simulink model "ASMC_sim_CSEI_FTESO"  (R2022a)
settings: Solver=ode4  StartTime=0.0  StopTime=T_final  FixedStep=Ts  RelTol=1e-3
values from neighbouring files (symbols this model uses):
  ASMC_enabled = 1    [ASMC_ESO_sim_CSEI_Scripts.m]    (also in ASMC_FTESO_sim_CSEI_Scripts.m)
  BL = [20 10 10]    [ASMC_ESO_sim_CSEI_Scripts.m]    (also in ASMC_FTESO_sim_CSEI_Scripts.m; SMC_ESO_sim_CSEI_Scripts.m; SMC_sim_CSEI_Scripts.m)
  Control_allocation = 1    [ASMC_ESO_sim_CSEI_Scripts.m]    (also in ASMC_FTESO_sim_CSEI_Scripts.m; SMC_ESO_sim_CSEI_Scripts.m; SMC_sim_CSEI_Scripts.m)
  current = [0;0]    [ASMC_ESO_sim_CSEI_Scripts.m]    (also in ASMC_FTESO_sim_CSEI_Scripts.m; Berthing_Control_PID_CSEI_Scripts.m; Position_Control_PID_CSEI_Scripts.m; Position_Control_PID_CSEI_Scripts_released.m)
  Disturbance_enabled = 1    [ASMC_ESO_sim_CSEI_Scripts.m]    (also in ASMC_FTESO_sim_CSEI_Scripts.m; SMC_ESO_sim_CSEI_Scripts.m)
  disturbance_type = 0    [ASMC_ESO_sim_CSEI_Scripts.m]    (also in ASMC_FTESO_sim_CSEI_Scripts.m = 2)
  ESO_enabled = 1    [ASMC_ESO_sim_CSEI_Scripts.m]    (also in ASMC_FTESO_sim_CSEI_Scripts.m; SMC_ESO_sim_CSEI_Scripts.m = 0)
  ESO_type = 2    [ASMC_FTESO_sim_CSEI_Scripts.m]
  ESO_type_enabled = 1    [ASMC_FTESO_sim_CSEI_Scripts.m]
  k1_init = 0.1*[5;5;10]    [ASMC_ESO_sim_CSEI_Scripts.m]    (also in ASMC_FTESO_sim_CSEI_Scripts.m)
  k2 = [5;5;5]    [ASMC_ESO_sim_CSEI_Scripts.m]    (also in ASMC_FTESO_sim_CSEI_Scripts.m)
  k3 = 0.05*[10; 20; 50]    [ASMC_ESO_sim_CSEI_Scripts.m]    (also in ASMC_FTESO_sim_CSEI_Scripts.m)
  k_min = 1    [ASMC_ESO_sim_CSEI_Scripts.m]    (also in ASMC_FTESO_sim_CSEI_Scripts.m)
  K_SMC = [20 20 50]    [ASMC_ESO_sim_CSEI_Scripts.m]    (also in ASMC_FTESO_sim_CSEI_Scripts.m; SMC_ESO_sim_CSEI_Scripts.m; SMC_sim_CSEI_Scripts.m)
  lamda = [5.0 5.0 10]    [ASMC_ESO_sim_CSEI_Scripts.m]    (also in ASMC_FTESO_sim_CSEI_Scripts.m; SMC_ESO_sim_CSEI_Scripts.m; SMC_sim_CSEI_Scripts.m)
  mu = [0.005; 0.005; 0.005]    [ASMC_ESO_sim_CSEI_Scripts.m]    (also in ASMC_FTESO_sim_CSEI_Scripts.m)
  option = 0    [ASMC_ESO_sim_CSEI_Scripts.m]    (also in ASMC_FTESO_sim_CSEI_Scripts.m; SMC_ESO_sim_CSEI_Scripts.m = 1; SMC_sim_CSEI_Scripts.m = 1)
  psi_ref = 40    [ASMC_ESO_sim_CSEI_Scripts.m]    (also in ASMC_FTESO_sim_CSEI_Scripts.m; SMC_ESO_sim_CSEI_Scripts.m; SMC_sim_CSEI_Scripts.m)
  tau_max = 20*[3; 3; 3]    [ASMC_ESO_sim_CSEI_Scripts.m]    (also in ASMC_FTESO_sim_CSEI_Scripts.m; SMC_ESO_sim_CSEI_Scripts.m; SMC_sim_CSEI_Scripts.m)
  v_max = 10    [ASMC_ESO_sim_CSEI_Scripts.m]    (also in ASMC_FTESO_sim_CSEI_Scripts.m; Position_Control_PID_CSEI_Scripts.m = 2; Position_Control_PID_CSEI_Scripts_released.m = 2; SMC_ESO_sim_CSEI_Scripts.m)
  w0 = 60    [ASMC_ESO_sim_CSEI_Scripts.m]    (also in ASMC_FTESO_sim_CSEI_Scripts.m; SMC_ESO_sim_CSEI_Scripts.m)
  w0_FTESO = 10    [ASMC_FTESO_sim_CSEI_Scripts.m]
  w_d = 0.5    [ASMC_ESO_sim_CSEI_Scripts.m]    (also in ASMC_FTESO_sim_CSEI_Scripts.m; SMC_ESO_sim_CSEI_Scripts.m; SMC_sim_CSEI_Scripts.m)
  x0 = zeros(6,1)    [Berthing_Control_PID_CSEI_Scripts.m]    (also in Position_Control_PID_CSEI_Scripts.m; Position_Control_PID_CSEI_Scripts_released.m; Waypoint_Control_PID_CSEI_Scripts.m; Waypoint_Control_PID_CSEI_Scripts_LLA.m)
  x_ref = 7    [ASMC_ESO_sim_CSEI_Scripts.m]    (also in ASMC_FTESO_sim_CSEI_Scripts.m; SMC_ESO_sim_CSEI_Scripts.m; SMC_sim_CSEI_Scripts.m)
  y_ref = 7    [ASMC_ESO_sim_CSEI_Scripts.m]    (also in ASMC_FTESO_sim_CSEI_Scripts.m; SMC_ESO_sim_CSEI_Scripts.m; SMC_sim_CSEI_Scripts.m)
  zeta_d = 1    [ASMC_ESO_sim_CSEI_Scripts.m]    (also in ASMC_FTESO_sim_CSEI_Scripts.m; SMC_ESO_sim_CSEI_Scripts.m; SMC_sim_CSEI_Scripts.m)
undefined symbols (not defined in the file or in its folder): sigbuilder_block
libraries: simulink_extras x5
(part 1 of 2)
settings Model: Creator=ADMIN  LastModifiedBy=ADMIN

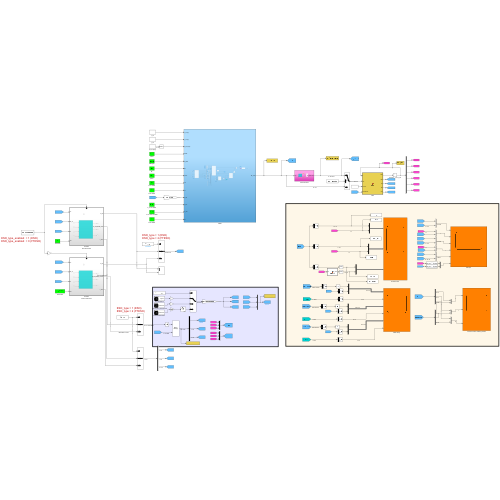
[thumbnail: Simulink's stored preview of the top-level diagram]
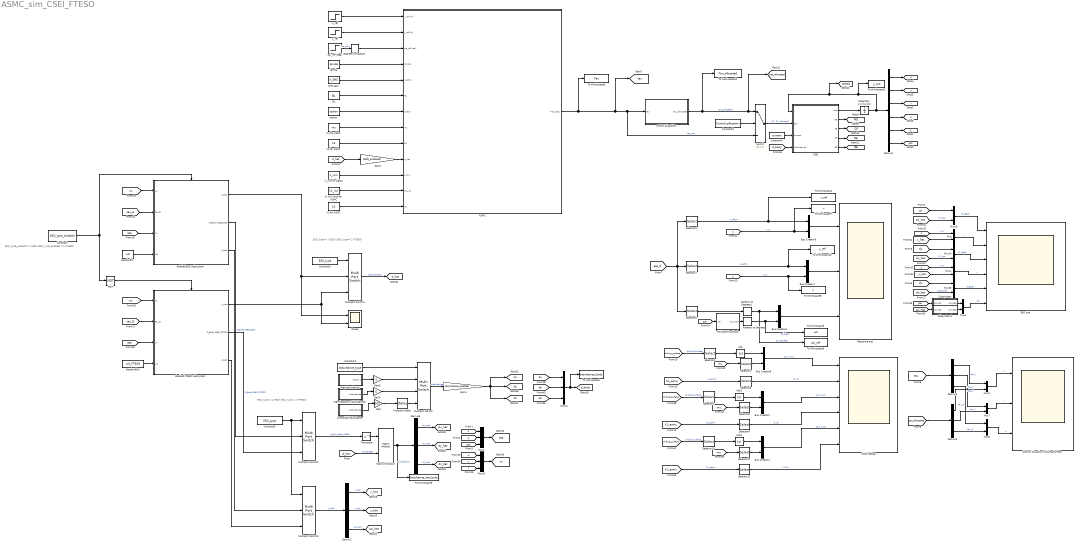
== system ASMC_sim_CSEI_FTESO ==
  note: ESO_type = 1 (ESO)
      | ESO_type = 2 (FTESO)
  note: ESO_type = 1 (ESO)
      | ESO_type = 2 (FTESO)
  note: ESO_type_enabled = 1 (ESO)
      | ESO_type_enabled = 0 (FTESO)
  ASMC : Subsystem
  ASMC debug : Scope  NumInputPorts=6
  Abs : Abs  SaturateOnIntegerOverflow=off
  Abs1 : Abs  SaturateOnIntegerOverflow=off
  Abs2 : Abs  SaturateOnIntegerOverflow=off
  BL : Constant  Value=BL
  Bandwidth : Constant  Value=w0
  Bandwidth2 : Constant  Value=w0_FTESO
  Bus Creator{1..6} (6 alike) : BusCreator  Inputs=2
  CSEI : MATLAB Function  TreatAsAtomicUnit=on
  Constant : Constant  Value=ESO_type_enabled
  Constant1 : Constant  Value=disturbance_type
  Constant2 : Constant  Value=ESO_type
  Constant3 : Constant  Value=Control_allocation
  Constant4 : Constant  Value=current
  Constant5 : Constant  Value=ESO_type
  Control Alocation & Sliding Surface : Scope  NumInputPorts=3
  Degrees to Radians : simulink_extras/Transformations/Degrees to Radians
  Demux1 : Demux  Outputs=6
  Demux{2..3,5,8} (4 alike) : Demux  Outputs=3
  ESO plot : Scope  NumInputPorts=6
  Enabled ESO Subsystem : Subsystem  TreatAsAtomicUnit=on
  Enabled FTESO Subsystem : Subsystem  TreatAsAtomicUnit=on
  Gain : Gain  Gain=100
  Gain1 : Gain  Gain=Disturbance_enabled
  Gain2 : Gain  Gain=ESO_enabled
  Gain3 : Gain  Gain=6
  Gain5 : Gain  Gain=5
  "Integrator : u;v;r;x;y;psi" : Integrator  InitialCondition=x0
  MATLAB Function3 : MATLAB Function  TreatAsAtomicUnit=on
  Matrix Multiply3 : Product  Multiplication=Matrix(*)
  Multiport Switch : MultiPortSwitch  SaturateOnIntegerOverflow=off  InputSameDT=off
  Multiport Switch1 : MultiPortSwitch  Inputs=2  SaturateOnIntegerOverflow=off  InputSameDT=off
  Multiport Switch2 : MultiPortSwitch  Inputs=2  SaturateOnIntegerOverflow=off  InputSameDT=off
  Multiport Switch3 : MultiPortSwitch  Inputs=2  SaturateOnIntegerOverflow=off  InputSameDT=off
  Mux{,1,3..4,7..8,14..16} (9 alike) : Mux  Inputs=2
  Mux10 : Mux  Inputs=3
  Mux11 : Mux  Inputs=3
  Mux2 : Mux  Inputs=3
  NOT : Logic  Operator=NOT  IconShape=distinctive  AllPortsSameDT=off  OutDataTypeStr=boolean
  Radians to Degrees : simulink_extras/Transformations/Radians to Degrees
  Radians to Degrees1 : simulink_extras/Transformations/Radians to Degrees
  Response plot : Scope  NumInputPorts=3
  SMC gain : Constant  Value=K_SMC
  Scope : Scope  NumInputPorts=2
  Selector1 : Selector  InputPortWidth=3  IndexOptions=Index vector (dialog)  Indices=1  OutputSizes=1
  Selector10 : Selector  InputPortWidth=3  IndexOptions=Index vector (dialog)  Indices=3  OutputSizes=1
  Selector11 : Selector  InputPortWidth=3  IndexOptions=Index vector (dialog)  Indices=3  OutputSizes=1
  Selector12 : Selector  InputPortWidth=3  IndexOptions=Index vector (dialog)  Indices=3  OutputSizes=1
  Selector2 : Selector  InputPortWidth=3  IndexOptions=Index vector (dialog)  Indices=1  OutputSizes=1
  Selector3 : Selector  InputPortWidth=3  IndexOptions=Index vector (dialog)  Indices=1  OutputSizes=1
  Selector4 : Selector  InputPortWidth=3  IndexOptions=Index vector (dialog)  Indices=2  OutputSizes=1
  Selector5 : Selector  InputPortWidth=3  IndexOptions=Index vector (dialog)  Indices=[3]  OutputSizes=1
  Selector6 : Selector  InputPortWidth=3  IndexOptions=Index vector (dialog)  Indices=[1]  OutputSizes=1
  Selector7 : Selector  InputPortWidth=3  IndexOptions=Index vector (dialog)  Indices=[2]  OutputSizes=1
  Selector8 : Selector  InputPortWidth=3  IndexOptions=Index vector (dialog)  Indices=2  OutputSizes=1
  Selector9 : Selector  InputPortWidth=3  IndexOptions=Index vector (dialog)  Indices=2  OutputSizes=1
  Subsystem : Subsystem
  Subsystem1 : Subsystem
  Switch : Switch  Criteria=u2 > Threshold  SaturateOnIntegerOverflow=off  InputSameDT=off
  To Workspace1 : ToWorkspace  VariableName=disturbance_body  SampleTime=-1
  To Workspace10 : ToWorkspace  VariableName=y_ref  SampleTime=-1
  To Workspace12 : ToWorkspace  VariableName=Tau_allocated  SampleTime=-1
  To Workspace2 : ToWorkspace  VariableName=y_out  SampleTime=-1
  To Workspace3 : ToWorkspace  VariableName=psi  SampleTime=-1
      settings: Save2DSignal=2-D array (concatenate along first dimension)
  To Workspace4 : ToWorkspace  VariableName=x_ref  SampleTime=-1
  To Workspace5 : ToWorkspace  VariableName=psi_ref  SampleTime=-1
  To Workspace6 : ToWorkspace  VariableName=Tau  SampleTime=-1
  To Workspace7 : ToWorkspace  VariableName=x  SampleTime=-1
      settings: Save2DSignal=2-D array (concatenate along first dimension)
  To Workspace8 : ToWorkspace  VariableName=y  SampleTime=-1
  To Workspace9 : ToWorkspace  VariableName=disturbance_hat_body  SampleTime=-1
  Transport Delay : TransportDelay  DelayTime=20
  Transpose : Math  Operator=transpose
  control allocation : Subsystem
  high-frequency disturbances : Subsystem  Tag=STV Subsys  LoadFcn=sigbuilder_block('load');  StartFcn=sigbuilder_block('start');  StopFcn=sigbuilder_block('stop');  ClipboardFcn=sigbuilder_block('clipboard');  mask(Sigbuilder block){tuvar=[0:10]}
      mask help: Simulink:masks:SigbuilderBlock_MD
      mask init:
      | if ~strcmp(get_param(bdroot(gcbh),'SimulationStatus'),'stopped') tuvar = sigbuilder_block('maskInit'); end
      settings: CopyFcn=sigbuilder_block('copy');  DeleteFcn=sigbuilder_block('delete');  ModelCloseFcn=sigbuilder_block('modelClose');  PreSaveFcn=sigbuilder_block('preSave');  PauseFcn=sigbuilder_block('pause');  ContinueFcn=sigbuilder_block('continue');  NameChangeFcn=sigbuilder_block('namechange');  OpenFcn=sigbuilder_block('open',[437.6 199.2 550.4 400 ]);  CloseFcn=sigbuilder_block('close');
      mask Display: plot(0, 0, 100, 100,[2, 2, 32, 32, 2], [68, 8, 8, 68, 68],[32, 2], [38, 38], [32, 19, 2],[53, 60, 44], [32, 17, 17, 2],[16, 16, 31, 31]);txt = getActiveGroup(gcbh);text(2, 100, txt,'verticalAlignment', 'top');
  k1 init value for ASMC : Constant  Value=k1_init
  k2 for ASMC : Constant  Value=k2
  k3 for ASMC : Constant  Value=k3
  k_min for ASMC : Constant  Value=k_min
  lamda : Constant  Value=lamda
  mu for ASMC : Constant  Value=mu
  option : Constant  Value=option
  psi_ref (deg) : Step  Time=10  After=psi_ref  SampleTime=0
  sinosoidal disturbance : Subsystem  Tag=STV Subsys  LoadFcn=sigbuilder_block('load');  StartFcn=sigbuilder_block('start');  StopFcn=sigbuilder_block('stop');  ClipboardFcn=sigbuilder_block('clipboard');  mask(Sigbuilder block){tuvar=[0:10]}
      mask help: Simulink:masks:SigbuilderBlock_MD
      mask init:
      | if ~strcmp(get_param(bdroot(gcbh),'SimulationStatus'),'stopped') tuvar = sigbuilder_block('maskInit'); end
      settings: CopyFcn=sigbuilder_block('copy');  DeleteFcn=sigbuilder_block('delete');  ModelCloseFcn=sigbuilder_block('modelClose');  PreSaveFcn=sigbuilder_block('preSave');  PauseFcn=sigbuilder_block('pause');  ContinueFcn=sigbuilder_block('continue');  NameChangeFcn=sigbuilder_block('namechange');  OpenFcn=sigbuilder_block('open',[437.6 199.2 550.4 400 ]);  CloseFcn=sigbuilder_block('close');
      mask Display: plot(0, 0, 100, 100,[2, 2, 32, 32, 2], [68, 8, 8, 68, 68],[32, 2], [38, 38], [32, 19, 2],[53, 60, 44], [32, 17, 17, 2],[16, 16, 31, 31]);txt = getActiveGroup(gcbh);text(2, 100, txt,'verticalAlignment', 'top');
  step disturbance : Subsystem  Tag=STV Subsys  LoadFcn=sigbuilder_block('load');  StartFcn=sigbuilder_block('start');  StopFcn=sigbuilder_block('stop');  ClipboardFcn=sigbuilder_block('clipboard');  mask(Sigbuilder block){tuvar=[0:10]}
      mask help: Simulink:masks:SigbuilderBlock_MD
      mask init:
      | if ~strcmp(get_param(bdroot(gcbh),'SimulationStatus'),'stopped') tuvar = sigbuilder_block('maskInit'); end
      settings: CopyFcn=sigbuilder_block('copy');  DeleteFcn=sigbuilder_block('delete');  ModelCloseFcn=sigbuilder_block('modelClose');  PreSaveFcn=sigbuilder_block('preSave');  PauseFcn=sigbuilder_block('pause');  ContinueFcn=sigbuilder_block('continue');  NameChangeFcn=sigbuilder_block('namechange');  OpenFcn=sigbuilder_block('open',[437.6 199.2 550.4 400 ]);  CloseFcn=sigbuilder_block('close');
      mask Display: plot(0, 0, 100, 100,[2, 2, 32, 32, 2], [68, 8, 8, 68, 68],[32, 2], [38, 38], [32, 19, 2],[53, 60, 44], [32, 17, 17, 2],[16, 16, 31, 31]);txt = getActiveGroup(gcbh);text(2, 100, txt,'verticalAlignment', 'top');
  x_ref : Step  Time=5  After=x_ref  SampleTime=0
  y_ref : Step  Time=5  After=y_ref  SampleTime=0
  tag scope: CE=global, DE=global, GE=global, ME=global, d_body=global, d_hat=global, dn=global, dn_hat=global, dx=global, dx_hat=global, dy=global, dy_hat=global, eta=global, nu=global, psi=global, psi_hat=global, r=global, states=global, tau=global, tau_allocated=global, u=global, v=global, x=global, x_hat=global, y=global, y_hat=global
  wires:
  Demux1/2 -> [v]
  Demux1/4 -> [x]
  Demux1/3 -> [r]
  CSEI/1(xdot) -> "Integrator : u;v;r;x;y;psi"/1
  Demux1/6 -> [psi]
  Demux1/1 -> [u]
  Demux1/5 -> [y]
  Constant3/1 -> Switch/2
  Constant4/1 -> CSEI/3(current)
  CSEI/2(ME) -> [ME]
  CSEI/3(CE) -> [CE]
  CSEI/4(DE) -> [DE]
  psi_ref (deg)/1 -> Degrees to Radians/1  "psi_ref"
  CSEI/5(GE) -> [GE]
  [x] -> Mux2/1
  [y] -> Mux2/2
  [psi] -> Mux2/3
  Mux2/1 -> [eta]
  "Integrator : u;v;r;x;y;psi"/1 -> To Workspace2/1, [states], CSEI/1(x), Demux1/1
  Switch/1 -> CSEI/2(tau)  "[Fx, Fy, Moment]"
  [tau] -> Demux3/1
  [tau_allocated] -> Demux5/1
  Mux3/1 -> Control Alocation & Sliding Surface/1  "X"
  Mux8/1 -> Control Alocation & Sliding Surface/3  "N"
  Demux3/1 -> Mux3/1  "tau_X"
  Demux3/2 -> Mux7/1  "tau_Y"
  Demux3/3 -> Mux8/1  "tau_N"
  Demux5/1 -> Mux3/2  "tau_X"
  Demux5/2 -> Mux7/2  "tau_Y"
  Demux5/3 -> Mux8/2  "tau_N"
  Mux7/1 -> Control Alocation & Sliding Surface/2  "Y"
  Gain1/1 -> [dn], [dy], [dx]
  Mux11/1 -> To Workspace1/1, [d_body]
  [dy] -> Mux11/2
  Gain/1 -> Transport Delay/1
  sinosoidal disturbance/1(disturbance) -> Gain/1
  [dn] -> Mux11/3
  [dx] -> Mux11/1
  Demux8/1 -> [dx_hat]  "dx_hat"
  Demux8/3 -> [dn_hat]  "dn_hat"
  Demux8/2 -> [dy_hat]  "dy_hat"
  Mux10/1 -> [nu]
  [u] -> Mux10/1
  [v] -> Mux10/2
  [r] -> Mux10/3
  Mux16/1 -> ESO plot/1  "Fx_Body"
  Matrix Multiply3/1 -> To Workspace9/1, Demux8/1  "d_hat_body"
  [dn_hat] -> Mux15/2  "N_dis_hat"
  [dy_hat] -> Mux14/2  "Fy_hat"
  [dx_hat] -> Mux16/2  "Fx_hat"
  [d_body] -> CSEI/4(disturbance)
  [d_hat] -> Gain2/1
  [mu] -> Selector2/1
  Bus Creator6/1 -> ASMC debug/1  "s1 & mu1"
  [sliding_surface] -> Selector1/1  "Sliding Surface"
  Abs/1 -> Bus Creator6/1
  Selector1/1 -> Abs/1
  Selector2/1 -> Bus Creator6/2
  [k1_asmc] -> Selector3/1  "k1_asmc"
  Selector3/1 -> ASMC debug/2  "k1 (1)"
  [sliding_surface] -> Selector4/1  "Sliding Surface"
  Selector4/1 -> Abs1/1
  [k1_asmc] -> Selector9/1  "k1_asmc"
  [mu] -> Selector8/1
  Abs1/1 -> Bus Creator2/1
  Bus Creator2/1 -> ASMC debug/3  "s2 & mu2"
  Selector9/1 -> ASMC debug/4  "k1 (2)"
  Selector8/1 -> Bus Creator2/2
  Bus Creator4/1 -> ASMC debug/5  "s3 & mu3"
  Abs2/1 -> Bus Creator4/1
  [k1_asmc] -> Selector12/1  "k1_asmc"
  [mu] -> Selector11/1
  Selector10/1 -> Abs2/1
  [sliding_surface] -> Selector10/1  "Sliding Surface"
  Selector12/1 -> ASMC debug/6  "k1 (3)"
  Selector11/1 -> Bus Creator4/2
  step disturbance/1(Signal 1) -> Gain5/1
  Constant1/1 -> Multiport Switch/1
  Multiport Switch/1 -> Gain1/1  "disturbances"
  Gain5/1 -> Multiport Switch/2
  ASMC/1(Tau_body) -> Switch/3, control allocation/1(tau), [tau], To Workspace6/1  "tau_raw"
  x_ref/1 -> ASMC/1(x_ref (m))
  y_ref/1 -> ASMC/2(y_ref (m))
  Degrees to Radians/1 -> ASMC/3(psi_ref (rad))
  lamda/1 -> ASMC/4(lamda)
  SMC gain/1 -> ASMC/5(K_SMC)
  BL/1 -> ASMC/6(BL)
  option/1 -> ASMC/7(option)
  mu for ASMC/1 -> ASMC/8(mu)
  k3 for ASMC/1 -> ASMC/9(k3)
  Gain2/1 -> ASMC/10(d_hat)
  k_min for ASMC/1 -> ASMC/11(k_min)
  k1 init value for ASMC/1 -> ASMC/12(k1_init)
  k2 for ASMC/1 -> ASMC/13(k2)
  control allocation/1(tau_allocated) -> [tau_allocated], Switch/1, To Workspace12/1  "tau_allocated"
  [nu] -> Enabled FTESO Subsystem/1(nu)
  [tau_E] -> Enabled FTESO Subsystem/2(tau_E)
  [eta] -> Enabled FTESO Subsystem/3(x1)
  Bandwidth2/1 -> Enabled FTESO Subsystem/4(w0)
  Radians to Degrees1/1 -> To Workspace5/1, Bus Creator3/1  "psi_ref_deg"
  Bus Creator3/1 -> Response plot/3
  MATLAB Function3/1(psi_mod) -> Radians to Degrees/1
  Radians to Degrees/1 -> Bus Creator3/2, To Workspace3/1  "psi_deg"
  [psi] -> MATLAB Function3/1(psi)
  Selector5/1 -> Radians to Degrees1/1
  Selector6/1 -> To Workspace4/1, Bus Creator5/1  "x_ref_m"
  Bus Creator5/1 -> Response plot/1
  [x] -> Bus Creator5/2, To Workspace7/1  "x_m"
  [eta_d] -> Selector5/1, Selector7/1, Selector6/1
  Selector7/1 -> To Workspace10/1, Bus Creator1/1  "y_ref_m"
  [y] -> To Workspace8/1, Bus Creator1/2  "y_m"
  Bus Creator1/1 -> Response plot/2
  [d_hat] -> Matrix Multiply3/2  "d_hat_NED"
  Transpose/1 -> Matrix Multiply3/1
  [dx] -> Mux16/1
  [dy] -> Mux14/1
  [dn] -> Mux15/1
  high-frequency disturbances/1(disturbance) -> Gain3/1
  Gain3/1 -> Multiport Switch/3
  Transport Delay/1 -> Multiport Switch/4
  Enabled FTESO Subsystem/1(d_hat) -> Multiport Switch1/3, Scope/2
  Enabled ESO Subsystem/1(d_hat) -> Scope/1, Multiport Switch1/2
  Constant2/1 -> Multiport Switch1/1
  Multiport Switch1/1 -> [d_hat]  "disturbances"
  [nu] -> Enabled ESO Subsystem/1(nu)
  [tau_E] -> Enabled ESO Subsystem/2(tau_E)
  [eta] -> Enabled ESO Subsystem/3(x1)
  Bandwidth/1 -> Enabled ESO Subsystem/4(w0)
  Constant/1 -> Enabled ESO Subsystem/Enable, NOT/1
  NOT/1 -> Enabled FTESO Subsystem/Enable
  Constant5/1 -> Multiport Switch3/1, Multiport Switch2/1
  Enabled ESO Subsystem/2(R_Body2NED_ESO) -> Multiport Switch2/2  "R_Body2NED_ESO"
  Enabled FTESO Subsystem/2(R_Body2NED_FTESO) -> Multiport Switch2/3  "R_Body2NED_FTESO"
  Multiport Switch2/1 -> Transpose/1  "R_from_Body2NED"
  Enabled FTESO Subsystem/3(x_hat1) -> Multiport Switch3/3
  Enabled ESO Subsystem/3(x_hat1) -> Multiport Switch3/2
  Demux2/1 -> [x_hat]  "x_hat"
  Demux2/3 -> [psi_hat]  "psi_hat"
  Demux2/2 -> [y_hat]  "y_hat"
  Multiport Switch3/1 -> Demux2/1  "x_hat1"
  Mux15/1 -> ESO plot/5  "N_Body"
  Mux14/1 -> ESO plot/3  "Fy_Body"
  Mux/1 -> ESO plot/2  "x"
  [x] -> Mux/1  "x_m"
  [y] -> Mux1/1  "x_m"
  Mux1/1 -> ESO plot/4  "y"
  Mux4/1 -> ESO plot/6  "psi"
  [psi] -> Subsystem/1(psi_rad)
  Subsystem/1(psi_deg) -> Mux4/1
  Subsystem1/1(psi_deg) -> Mux4/2
  [psi_hat] -> Subsystem1/1(psi_rad)
  [x_hat] -> Mux/2
  [y_hat] -> Mux1/2

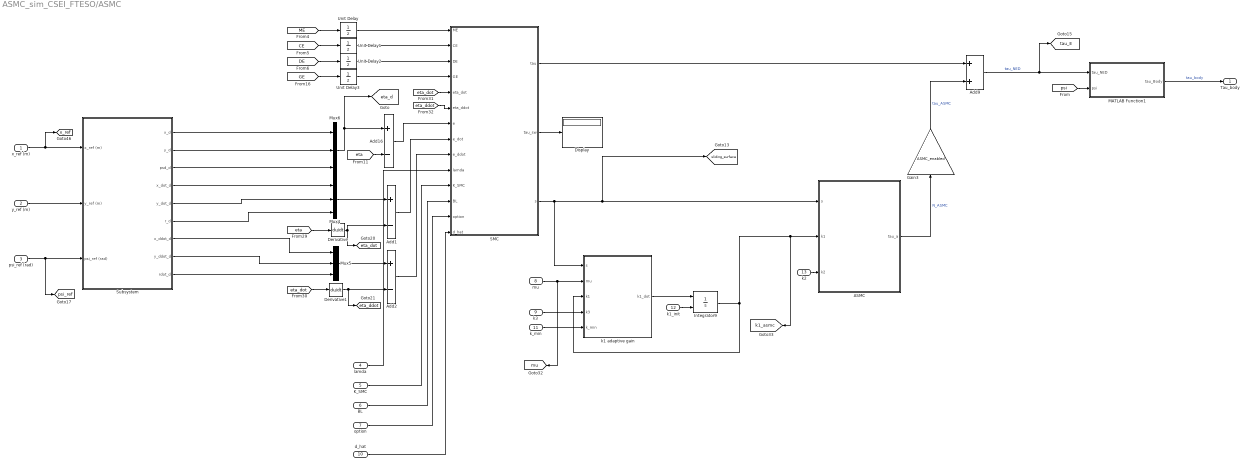
== system ASMC_sim_CSEI_FTESO/ASMC ==
  x_ref (m) : Inport
  y_ref (m) : Inport  Port=2
  psi_ref (rad) : Inport  Port=3
  lamda : Inport  Port=4
  K_SMC : Inport  Port=5
  BL : Inport  Port=6
  option : Inport  Port=7
  mu : Inport  Port=8
  k3 : Inport  Port=9
  d_hat : Inport  Port=10
  k_min : Inport  Port=11
  k1_init : Inport  Port=12
  k2 : Inport  Port=13
  ASMC : MATLAB Function  TreatAsAtomicUnit=on
  Add1 : Sum  Inputs=+-
  Add16 : Sum  Inputs=+-
  Add2 : Sum  Inputs=+-
  Add9 : Sum
  Derivative : Derivative
  Derivative1 : Derivative
  Display : Display
  Gain3 : Gain  Gain=ASMC_enabled
  Integrator9 : Integrator  InitialConditionSource=external  InitialCondition=0.01
  MATLAB Function1 : MATLAB Function  TreatAsAtomicUnit=on
  Mux4 : Mux  Inputs=3
  Mux5 : Mux  Inputs=3
  Mux6 : Mux  Inputs=3
  SMC : MATLAB Function  TreatAsAtomicUnit=on
  Subsystem : Subsystem
  Unit Delay{,1..3} (4 alike) : UnitDelay  SampleTime=-1  HasFrameUpgradeWarning=on
  k1 adaptive gain : MATLAB Function  TreatAsAtomicUnit=on
  Tau_body : Outport
  tag scope: eta_d=global, eta_ddot=global, eta_dot=global, k1_asmc=global, mu=global, psi_ref=global, sliding_surface=global, tau_E=global, x_ref=global
  wires:
  Integrator9/1 -> k1 adaptive gain/3(k1), ASMC/2(k1), [k1_asmc]
  [psi] -> MATLAB Function1/2(psi)
  Gain3/1 -> Add9/2  "tau_ASMC"
  [CE] -> Unit Delay1/1
  Mux5/1 -> Add2/1
  Subsystem/7(x_ddot_d) -> Mux5/1
  Add2/1 -> SMC/9(e_ddot)
  Derivative/1 -> [eta_dot], Add1/2
  Subsystem/8(y_ddot_d) -> Mux5/2
  [GE] -> Unit Delay3/1
  k3/1 -> k1 adaptive gain/4(k3)
  Subsystem/3(psd_d) -> Mux6/3
  [eta_dot] -> SMC/5(eta_dot)
  mu/1 -> [mu], k1 adaptive gain/2(mu)
  psi_ref (rad)/1 -> Subsystem/3(psi_ref (rad)), [psi_ref]
  Subsystem/1(x_d) -> Mux6/1
  Add16/1 -> SMC/7(e)
  Subsystem/2(y_d) -> Mux6/2
  [eta] -> Add16/2
  d_hat/1 -> SMC/14(d_hat)
  Derivative1/1 -> [eta_ddot], Add2/2
  SMC/3(s) -> [sliding_surface], ASMC/1(s), k1 adaptive gain/1(s)
  [ME] -> Unit Delay/1
  Unit Delay2/1 -> SMC/3(DE)
  k1 adaptive gain/1(k1_dot) -> Integrator9/1
  [DE] -> Unit Delay2/1
  Unit Delay/1 -> SMC/1(ME)
  [eta_dot] -> Derivative1/1
  Subsystem/5(y_dot_d) -> Mux4/2
  k1_init/1 -> Integrator9/2
  Add1/1 -> SMC/8(e_dot)
  BL/1 -> SMC/12(BL)
  ASMC/1(tau_a) -> Gain3/1  "N_ASMC"
  Unit Delay3/1 -> SMC/4(GE)
  k2/1 -> ASMC/3(k2)
  Subsystem/4(x_dot_d) -> Mux4/1
  Subsystem/9(rdot_d) -> Mux5/3
  Mux6/1 -> Add16/1, [eta_d]
  [eta_ddot] -> SMC/6(eta_ddot)
  y_ref (m)/1 -> Subsystem/2(y_ref (m))
  [eta] -> Derivative/1
  Add9/1 -> [tau_E], MATLAB Function1/1(tau_NED)  "tau_NED"
  option/1 -> SMC/13(option)
  Unit Delay1/1 -> SMC/2(CE)
  Mux4/1 -> Add1/1
  Subsystem/6(r_d) -> Mux4/3
  x_ref (m)/1 -> [x_ref], Subsystem/1(x_ref (m))
  SMC/2(tau_sw) -> Display/1
  SMC/1(tau) -> Add9/1
  K_SMC/1 -> SMC/11(K_SMC)
  lamda/1 -> SMC/10(lamda)
  k_min/1 -> k1 adaptive gain/5(k_min)
  MATLAB Function1/1(tau_Body) -> Tau_body/1  "tau_body"

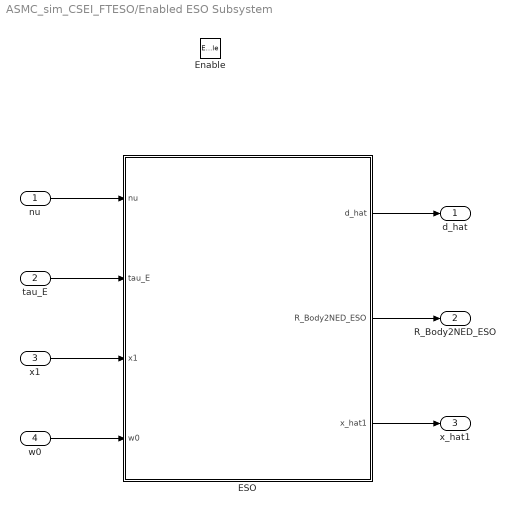
== system ASMC_sim_CSEI_FTESO/Enabled ESO Subsystem ==
  nu : Inport
  tau_E : Inport  Port=2
  x1 : Inport  Port=3
  w0 : Inport  Port=4
  Enable : EnablePort
  ESO : Subsystem
  d_hat : Outport
  R_Body2NED_ESO : Outport  Port=2
  x_hat1 : Outport  Port=3
  wires:
  ESO/1(d_hat) -> d_hat/1
  nu/1 -> ESO/1(nu)
  tau_E/1 -> ESO/2(tau_E)
  x1/1 -> ESO/3(x1)
  w0/1 -> ESO/4(w0)
  ESO/2(R_Body2NED_ESO) -> R_Body2NED_ESO/1
  ESO/3(x_hat1) -> x_hat1/1

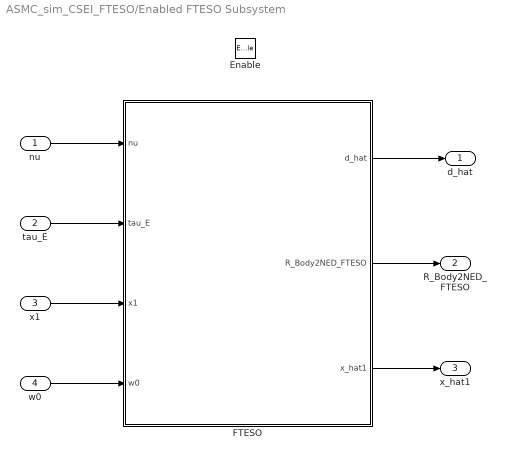
== system ASMC_sim_CSEI_FTESO/Enabled FTESO Subsystem ==
  nu : Inport
  tau_E : Inport  Port=2
  x1 : Inport  Port=3
  w0 : Inport  Port=4
  Enable : EnablePort
  FTESO : Subsystem
  d_hat : Outport
  R_Body2NED_FTESO : Outport  Port=2
  x_hat1 : Outport  Port=3
  wires:
  FTESO/1(d_hat) -> d_hat/1
  nu/1 -> FTESO/1(nu)
  tau_E/1 -> FTESO/2(tau_E)
  x1/1 -> FTESO/3(x1)
  w0/1 -> FTESO/4(w0)
  FTESO/2(R_Body2NED_FTESO) -> R_Body2NED_FTESO/1
  FTESO/3(x_hat1) -> x_hat1/1

== system ASMC_sim_CSEI_FTESO/Subsystem ==
  psi_rad : Inport
  MATLAB Function1 : MATLAB Function  TreatAsAtomicUnit=on
  Radians to Degrees2 : simulink_extras/Transformations/Radians to Degrees
  psi_deg : Outport
  wires:
  MATLAB Function1/1(psi_mod) -> Radians to Degrees2/1
  psi_rad/1 -> MATLAB Function1/1(psi)
  Radians to Degrees2/1 -> psi_deg/1  "psi"

== system ASMC_sim_CSEI_FTESO/Subsystem1 ==
  psi_rad : Inport
  MATLAB Function1 : MATLAB Function  TreatAsAtomicUnit=on
  Radians to Degrees2 : simulink_extras/Transformations/Radians to Degrees
  psi_deg : Outport
  wires:
  MATLAB Function1/1(psi_mod) -> Radians to Degrees2/1
  psi_rad/1 -> MATLAB Function1/1(psi)
  Radians to Degrees2/1 -> psi_deg/1  "psi"

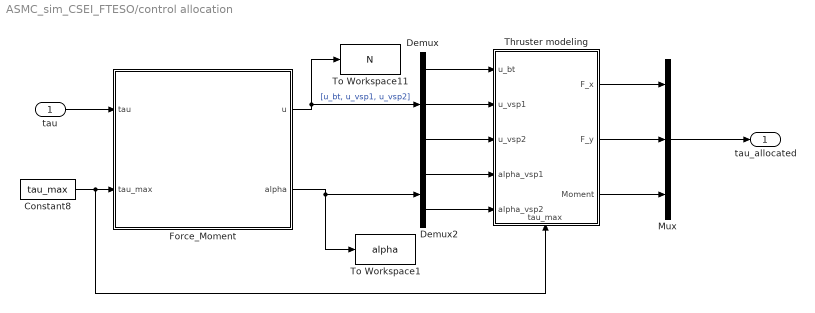
== system ASMC_sim_CSEI_FTESO/control allocation ==
  tau : Inport
  Constant8 : Constant  Value=tau_max
  Demux : Demux  Outputs=3
  Demux2 : Demux  Outputs=2
  Force_Moment : MATLAB Function  TreatAsAtomicUnit=on
  Mux : Mux  Inputs=3
  Thruster modeling : Subsystem
      settings: PortSchema="{\"entries\":[{\"content\":{\"sides\":[{\"content\":{\"connectorIds\":[\"In1\",\"In2\",\"In3\",\"In4\",\"In5\"]},\"type\":\"ConnectorPlacement.EquallySpacedRectSide\",\"uuid\":\"a9c62c9e-2a2a-45d5-affb-b7e02571c4f5\"},{\"content\":{\"connectorIds\":[\"Out1\",\"Out2\",\"Out3\"],\"side\":\"RIGHT\"},\"type\":\"ConnectorPlacement.EquallySpacedRectSide\",\"uuid\":\"bfdff314-1a15-4488-bfde-1b5f82948245\"},{\"content\":{\"connectorIds\":[],\"side\":\"TOP\"},\"type\":\"ConnectorPlacement.EquallySpacedRectSide\",\"uuid\":\"bddef62a-91eb-4612-9a88-29ec8ace0b5e\"},{\"content\":{\"connectorIds\":[\"In6\"],\"side\":\"BOTTOM\"},\"type\":\"ConnectorPlacement.EquallySpacedRectSide\",\"uuid\":\"97d017d6-0e26-4257-956b-3bb507a639f3\"}]},\"type\":\"ConnectorPlacement.EquallySpacedConnector\",\"uuid\":\"a9966a75-95cf-4066-83e4-2624c4c1c778\"}],\"packageUris\":[\"http://schema.mathworks.com/mf0/Connector/R2020b\"],\"version\":\"1.0\"}"
  To Workspace1 : ToWorkspace  VariableName=alpha  SampleTime=-1
  To Workspace11 : ToWorkspace  VariableName=N  SampleTime=-1
  tau_allocated : Outport
  wires:
  Thruster modeling/1(F_x) -> Mux/1
  Demux/2 -> Thruster modeling/2(u_vsp1)
  Demux2/1 -> Thruster modeling/4(alpha_vsp1)
  Force_Moment/1(u) -> To Workspace11/1, Demux/1  "[u_bt, u_vsp1, u_vsp2]"
  Demux/3 -> Thruster modeling/3("u_vsp2 ")
  Force_Moment/2(alpha) -> To Workspace1/1, Demux2/1
  Constant8/1 -> Thruster modeling/6(tau_max), Force_Moment/2(tau_max)
  Thruster modeling/2(F_y) -> Mux/2
  Thruster modeling/3("Moment ") -> Mux/3
  tau/1 -> Force_Moment/1(tau)
  Demux2/2 -> Thruster modeling/5(alpha_vsp2)
  Demux/1 -> Thruster modeling/1(u_bt)
  Mux/1 -> tau_allocated/1

== system ASMC_sim_CSEI_FTESO/high-frequency disturbances ==
  Demux : Demux  Tag=STV Demux  Outputs=1
      settings: DisplayOption=none
  FromWs : FromWorkspace  Tag=STV FromWs  VariableName=tuvar
      SigBuilderData=|
      | common.afterFinalStr = 'Extrapolate'
      | common.sampleTime = 0
      | dataSet.timeRange = [0 100]
      | dataSet.name = 'Sheet1'
      | sbobj.Groups.Name = 'Sheet1'
      | sbobj.Groups.Signals.Name = 'disturbance'
      | sbobj.Groups.Signals.XData = [0 0.0100010001 0.0200020002 0.0300030003 0.0400040004 0.0500050005001 0.0600060006001 0.0700070007001 0.0800080008001 0.0900090009001 0.100010001 0.1100110011 ... (10000 elements, 1x10000)]
      | sbobj.Groups.Signals.YData = [-0.00992566591604 -0.00860639120336 -0.00736343338162 -0.0061969124364 -0.00510679163825 -0.00409289174578 -0.00315490534947 -0.00229241123517 -0.00150488864817 -0.000791731342143 -0.000152261301172 0.000414257972155 ... (10000 elements, 1x10000)]
      | sbobj.Groups.TimeRange = [0 100]
  disturbance : Outport  Tag=STV Outport
  wires:
  Demux/1 -> disturbance/1
  FromWs/1 -> Demux/1

== system ASMC_sim_CSEI_FTESO/sinosoidal disturbance ==
  Demux : Demux  Tag=STV Demux  Outputs=1
      settings: DisplayOption=none
  FromWs : FromWorkspace  Tag=STV FromWs  VariableName=tuvar
      SigBuilderData=|
      | common.afterFinalStr = 'Extrapolate'
      | common.sampleTime = 0
      | dataSet.timeRange = [0 100]
      | dataSet.name = 'Sheet1'
      | sbobj.Groups.Name = 'Sheet1'
      | sbobj.Groups.Signals.Name = 'disturbance'
      | sbobj.Groups.Signals.XData = [0 0.0100010001 0.0200020002 0.0300030003 0.0400040004 0.0500050005001 0.0600060006001 0.0700070007001 0.0800080008001 0.0900090009001 0.100010001 0.1100110011 ... (10000 elements, 1x10000)]
      | sbobj.Groups.Signals.YData = [-0.00992566591604 -0.00860639120336 -0.00736343338162 -0.0061969124364 -0.00510679163825 -0.00409289174578 -0.00315490534947 -0.00229241123517 -0.00150488864817 -0.000791731342143 -0.000152261301172 0.000414257972155 ... (10000 elements, 1x10000)]
      | sbobj.Groups.TimeRange = [0 100]
  disturbance : Outport  Tag=STV Outport
  wires:
  Demux/1 -> disturbance/1
  FromWs/1 -> Demux/1

== system ASMC_sim_CSEI_FTESO/step disturbance ==
  Demux : Demux  Tag=STV Demux  Outputs=1
      settings: DisplayOption=none
  FromWs : FromWorkspace  Tag=STV FromWs  VariableName=tuvar
      SigBuilderData=|
      | common.afterFinalStr = 'Extrapolate'
      | common.sampleTime = 0
      | dataSet.timeRange = [0 100]
      | dataSet.name = 'Group 1'
      | sbobj.Groups.Name = 'Group 1'
      | sbobj.Groups.Signals.Name = 'Signal 1'
      | sbobj.Groups.Signals.XData = [0 40.4 40.4 60.4 60.4 100]
      | sbobj.Groups.Signals.YData = [0 0 1 1 0 0]
      | sbobj.Groups.TimeRange = [0 100]
  Signal 1 : Outport  Tag=STV Outport
  wires:
  Demux/1 -> Signal 1/1
  FromWs/1 -> Demux/1

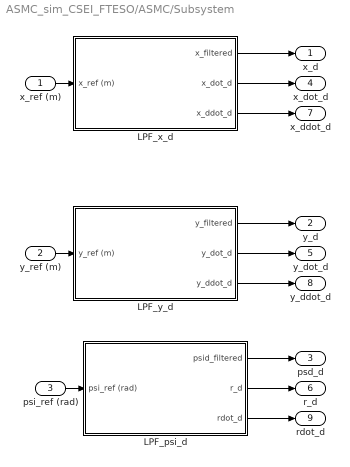
== system ASMC_sim_CSEI_FTESO/ASMC/Subsystem ==
  x_ref (m) : Inport
  y_ref (m) : Inport  Port=2
  psi_ref (rad) : Inport  Port=3
  LPF_psi_d : Subsystem
  LPF_x_d : Subsystem
  LPF_y_d : Subsystem
  x_d : Outport
  y_d : Outport  Port=2
  psd_d : Outport  Port=3
  x_dot_d : Outport  Port=4
  y_dot_d : Outport  Port=5
  r_d : Outport  Port=6
  x_ddot_d : Outport  Port=7
  y_ddot_d : Outport  Port=8
  rdot_d : Outport  Port=9
  wires:
  LPF_x_d/3(x_ddot_d) -> x_ddot_d/1
  LPF_x_d/2(x_dot_d) -> x_dot_d/1
  LPF_y_d/1(y_filtered) -> y_d/1
  x_ref (m)/1 -> LPF_x_d/1(x_ref (m))
  psi_ref (rad)/1 -> LPF_psi_d/1(psi_ref (rad))
  LPF_y_d/2(y_dot_d) -> y_dot_d/1
  LPF_x_d/1(x_filtered) -> x_d/1
  LPF_psi_d/2(r_d) -> r_d/1
  y_ref (m)/1 -> LPF_y_d/1(y_ref (m))
  LPF_psi_d/1(psid_filtered) -> psd_d/1
  LPF_psi_d/3(rdot_d) -> rdot_d/1
  LPF_y_d/3(y_ddot_d) -> y_ddot_d/1

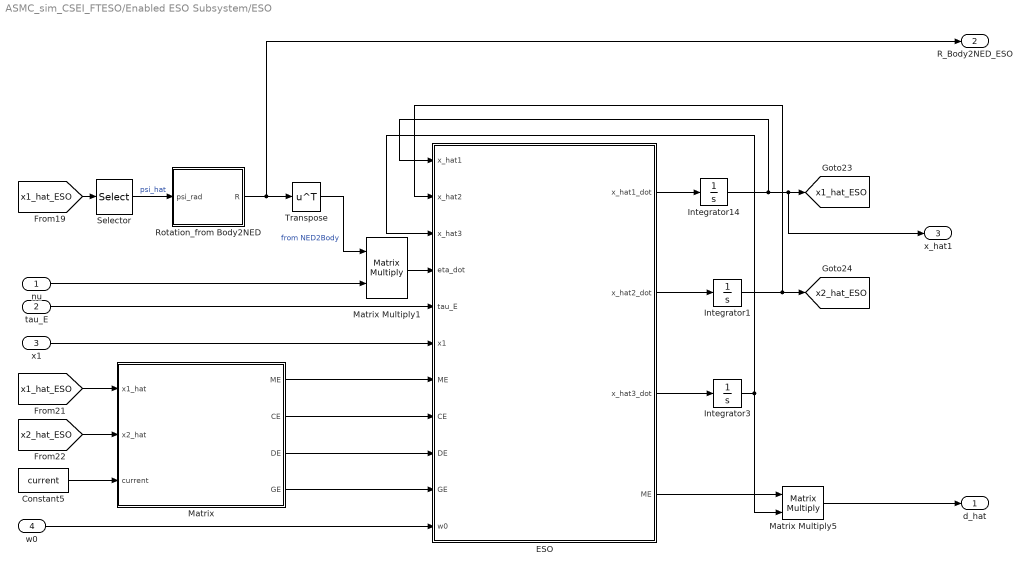
== system ASMC_sim_CSEI_FTESO/Enabled ESO Subsystem/ESO ==
  nu : Inport
  tau_E : Inport  Port=2
  x1 : Inport  Port=3
  w0 : Inport  Port=4
  Constant5 : Constant  Value=current
  ESO : MATLAB Function  TreatAsAtomicUnit=on
  Integrator1 : Integrator  InitialCondition=zeros(3,1)
  Integrator14 : Integrator  InitialCondition=zeros(3,1)
  Integrator3 : Integrator  InitialCondition=zeros(3,1)
  Matrix : MATLAB Function  TreatAsAtomicUnit=on
  Matrix Multiply1 : Product  Multiplication=Matrix(*)
  Matrix Multiply5 : Product  Multiplication=Matrix(*)
  Rotation_from Body2NED : Subsystem
  Selector : Selector  InputPortWidth=3  IndexOptions=Index vector (dialog)  Indices=3  OutputSizes=1
  Transpose : Math  Operator=transpose
  d_hat : Outport
  R_Body2NED_ESO : Outport  Port=2
  x_hat1 : Outport  Port=3
  tag scope: x1_hat_ESO=global, x2_hat_ESO=global
  wires:
  Integrator1/1 -> [x2_hat_ESO], ESO/2(x_hat2)
  Integrator14/1 -> x_hat1/1, [x1_hat_ESO], ESO/1(x_hat1)
  Transpose/1 -> Matrix Multiply1/1  "from NED2Body"
  Matrix/4(GE) -> ESO/10(GE)
  [x1_hat_ESO] -> Matrix/1(x1_hat)
  ESO/2(x_hat2_dot) -> Integrator1/1
  tau_E/1 -> ESO/5(tau_E)
  Matrix Multiply1/1 -> ESO/4(eta_dot)
  ESO/4(ME) -> Matrix Multiply5/1
  Constant5/1 -> Matrix/3(current)
  Selector/1 -> Rotation_from Body2NED/1(psi_rad)  "psi_hat"
  Rotation_from Body2NED/1(R) -> R_Body2NED_ESO/1, Transpose/1
  nu/1 -> Matrix Multiply1/2
  [x2_hat_ESO] -> Matrix/2(x2_hat)
  Matrix/2(CE) -> ESO/8(CE)
  Matrix/3(DE) -> ESO/9(DE)
  ESO/1(x_hat1_dot) -> Integrator14/1
  Integrator3/1 -> ESO/3(x_hat3), Matrix Multiply5/2
  ESO/3(x_hat3_dot) -> Integrator3/1
  Matrix/1(ME) -> ESO/7("ME ")
  [x1_hat_ESO] -> Selector/1
  w0/1 -> ESO/11(w0)
  Matrix Multiply5/1 -> d_hat/1
  x1/1 -> ESO/6(x1)

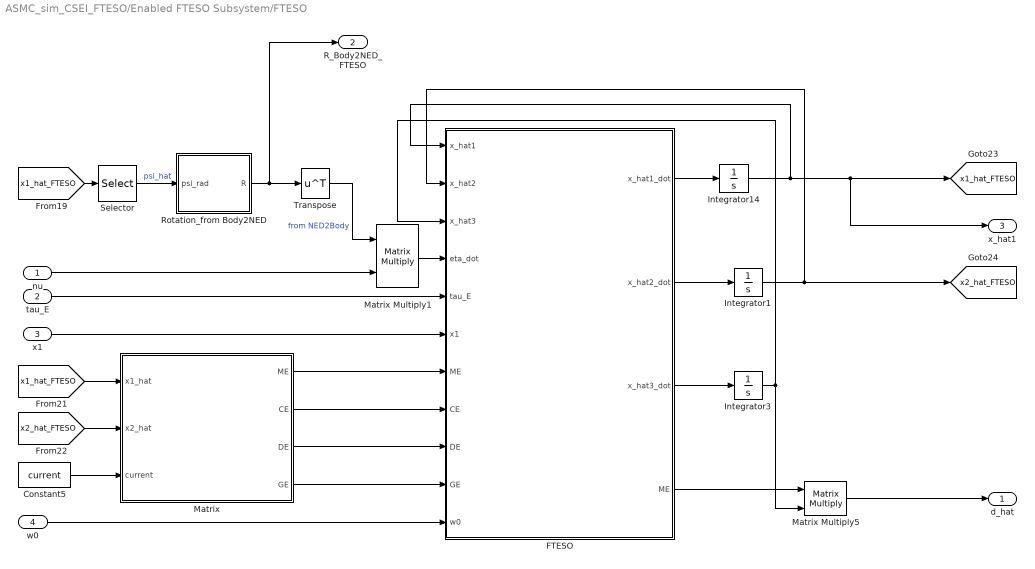
== system ASMC_sim_CSEI_FTESO/Enabled FTESO Subsystem/FTESO ==
  nu : Inport
  tau_E : Inport  Port=2
  x1 : Inport  Port=3
  w0 : Inport  Port=4
  Constant5 : Constant  Value=current
  FTESO : MATLAB Function  TreatAsAtomicUnit=on
  Integrator1 : Integrator  InitialCondition=zeros(3,1)
  Integrator14 : Integrator  InitialCondition=zeros(3,1)
  Integrator3 : Integrator  InitialCondition=zeros(3,1)
  Matrix : MATLAB Function  TreatAsAtomicUnit=on
  Matrix Multiply1 : Product  Multiplication=Matrix(*)
  Matrix Multiply5 : Product  Multiplication=Matrix(*)
  Rotation_from Body2NED : Subsystem
  Selector : Selector  InputPortWidth=3  IndexOptions=Index vector (dialog)  Indices=3  OutputSizes=1
  Transpose : Math  Operator=transpose
  d_hat : Outport
  R_Body2NED_FTESO : Outport  Port=2
  x_hat1 : Outport  Port=3
  tag scope: x1_hat_FTESO=global, x2_hat_FTESO=global
  wires:
  Integrator1/1 -> [x2_hat_FTESO], FTESO/2(x_hat2)
  Transpose/1 -> Matrix Multiply1/1  "from NED2Body"
  Matrix/4(GE) -> FTESO/10(GE)
  [x1_hat_FTESO] -> Matrix/1(x1_hat)
  FTESO/2(x_hat2_dot) -> Integrator1/1
  tau_E/1 -> FTESO/5(tau_E)
  Matrix Multiply1/1 -> FTESO/4(eta_dot)
  FTESO/4(ME) -> Matrix Multiply5/1
  Constant5/1 -> Matrix/3(current)
  Selector/1 -> Rotation_from Body2NED/1(psi_rad)  "psi_hat"
  Rotation_from Body2NED/1(R) -> R_Body2NED_FTESO/1, Transpose/1
  nu/1 -> Matrix Multiply1/2
  [x2_hat_FTESO] -> Matrix/2(x2_hat)
  Matrix/2(CE) -> FTESO/8(CE)
  Matrix/3(DE) -> FTESO/9(DE)
  FTESO/1(x_hat1_dot) -> Integrator14/1
  Integrator3/1 -> FTESO/3(x_hat3), Matrix Multiply5/2
  FTESO/3(x_hat3_dot) -> Integrator3/1
  Matrix/1(ME) -> FTESO/7("ME ")
  [x1_hat_FTESO] -> Selector/1
  w0/1 -> FTESO/11(w0)
  Matrix Multiply5/1 -> d_hat/1
  x1/1 -> FTESO/6(x1)
  Integrator14/1 -> x_hat1/1, [x1_hat_FTESO], FTESO/1(x_hat1)

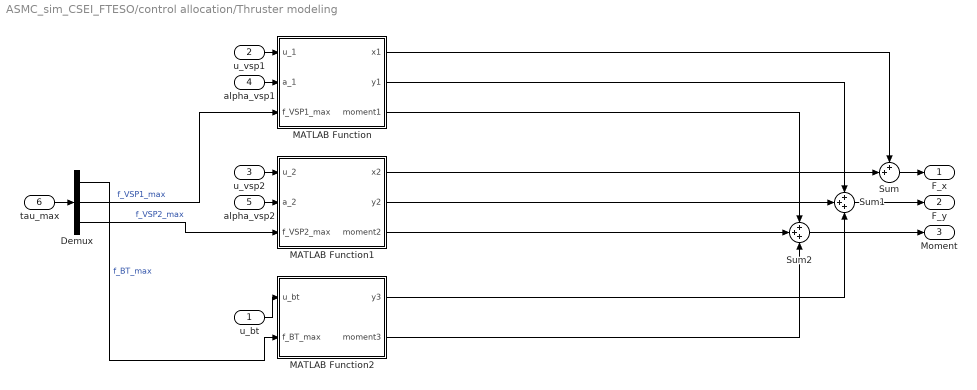
== system ASMC_sim_CSEI_FTESO/control allocation/Thruster modeling ==
  u_bt : Inport
  u_vsp1 : Inport  Port=2
  "u_vsp2 " : Inport  Port=3
  alpha_vsp1 : Inport  Port=4
  alpha_vsp2 : Inport  Port=5
  tau_max : Inport  Port=6
  Demux : Demux  Outputs=3
  MATLAB Function : MATLAB Function  TreatAsAtomicUnit=on
  MATLAB Function1 : MATLAB Function  TreatAsAtomicUnit=on
  MATLAB Function2 : MATLAB Function  TreatAsAtomicUnit=on
  Sum : Sum  Inputs=++|
  Sum1 : Sum  Inputs=+++
  Sum2 : Sum  Inputs=+++
  F_x : Outport
  F_y : Outport  Port=2
  "Moment " : Outport  Port=3
  wires:
  u_bt/1 -> MATLAB Function2/1(u_bt)
  alpha_vsp2/1 -> MATLAB Function1/2(a_2)
  u_vsp1/1 -> MATLAB Function/1(u_1)
  "u_vsp2 "/1 -> MATLAB Function1/1(u_2)
  MATLAB Function1/1(x2) -> Sum/2
  Sum/1 -> F_x/1
  Sum1/1 -> F_y/1
  MATLAB Function1/2(y2) -> Sum1/2
  MATLAB Function2/1(y3) -> Sum1/3
  Sum2/1 -> "Moment "/1
  MATLAB Function2/2(moment3) -> Sum2/3
  MATLAB Function1/3(moment2) -> Sum2/2
  MATLAB Function/3(moment1) -> Sum2/1
  MATLAB Function/1(x1) -> Sum/1
  MATLAB Function/2(y1) -> Sum1/1
  tau_max/1 -> Demux/1
  Demux/1 -> MATLAB Function2/2(f_BT_max)  "f_BT_max"
  alpha_vsp1/1 -> MATLAB Function/2(a_1)
  Demux/2 -> MATLAB Function/3(f_VSP1_max)  "f_VSP1_max"
  Demux/3 -> MATLAB Function1/3(f_VSP2_max)  "f_VSP2_max"

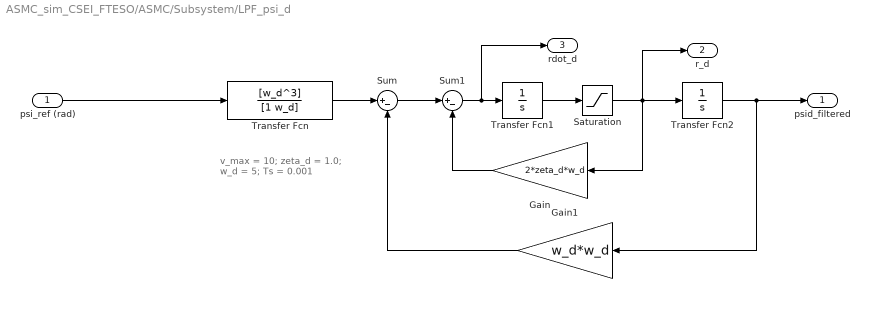
== system ASMC_sim_CSEI_FTESO/ASMC/Subsystem/LPF_psi_d ==
  note: v_max = 10;
      | zeta_d = 1.0;
      | w_d = 5;
      | Ts = 0.001
  psi_ref (rad) : Inport
  Gain : Gain  Gain=2*zeta_d*w_d
  Gain1 : Gain  Gain=w_d*w_d
  Saturation : Saturate  UpperLimit=v_max  LowerLimit=-v_max  LinearizeAsGain=off
  Sum : Sum  Inputs=|+-
  Sum1 : Sum  Inputs=|+-
  Transfer Fcn : TransferFcn  Numerator=[w_d^3]  Denominator=[1 w_d]
  Transfer Fcn1 : TransferFcn  Denominator=[1 0]
  Transfer Fcn2 : TransferFcn  Denominator=[1 0]
  psid_filtered : Outport
  r_d : Outport  Port=2
  rdot_d : Outport  Port=3
  wires:
  Transfer Fcn/1 -> Sum/1
  Transfer Fcn1/1 -> Saturation/1
  Sum1/1 -> rdot_d/1, Transfer Fcn1/1
  Saturation/1 -> r_d/1, Gain/1, Transfer Fcn2/1
  Gain1/1 -> Sum/2
  Sum/1 -> Sum1/1
  Transfer Fcn2/1 -> psid_filtered/1, Gain1/1
  Gain/1 -> Sum1/2
  psi_ref (rad)/1 -> Transfer Fcn/1

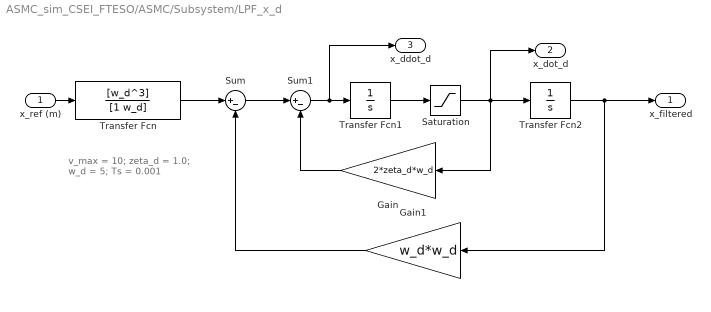
== system ASMC_sim_CSEI_FTESO/ASMC/Subsystem/LPF_x_d ==
  note: v_max = 10;
      | zeta_d = 1.0;
      | w_d = 5;
      | Ts = 0.001
  x_ref (m) : Inport
  Gain : Gain  Gain=2*zeta_d*w_d
  Gain1 : Gain  Gain=w_d*w_d
  Saturation : Saturate  UpperLimit=v_max  LowerLimit=-v_max  LinearizeAsGain=off
  Sum : Sum  Inputs=|+-
  Sum1 : Sum  Inputs=|+-
  Transfer Fcn : TransferFcn  Numerator=[w_d^3]  Denominator=[1 w_d]
  Transfer Fcn1 : TransferFcn  Denominator=[1 0]
  Transfer Fcn2 : TransferFcn  Denominator=[1 0]
  x_filtered : Outport
  x_dot_d : Outport  Port=2
  x_ddot_d : Outport  Port=3
  wires:
  Transfer Fcn/1 -> Sum/1
  Transfer Fcn1/1 -> Saturation/1
  Sum1/1 -> x_ddot_d/1, Transfer Fcn1/1
  Saturation/1 -> x_dot_d/1, Gain/1, Transfer Fcn2/1
  Gain1/1 -> Sum/2
  Sum/1 -> Sum1/1
  Transfer Fcn2/1 -> x_filtered/1, Gain1/1
  Gain/1 -> Sum1/2
  x_ref (m)/1 -> Transfer Fcn/1

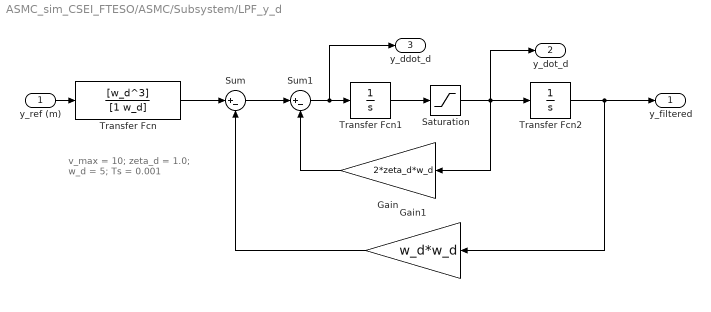
== system ASMC_sim_CSEI_FTESO/ASMC/Subsystem/LPF_y_d ==
  note: v_max = 10;
      | zeta_d = 1.0;
      | w_d = 5;
      | Ts = 0.001
  y_ref (m) : Inport
  Gain : Gain  Gain=2*zeta_d*w_d
  Gain1 : Gain  Gain=w_d*w_d
  Saturation : Saturate  UpperLimit=v_max  LowerLimit=-v_max  LinearizeAsGain=off
  Sum : Sum  Inputs=|+-
  Sum1 : Sum  Inputs=|+-
  Transfer Fcn : TransferFcn  Numerator=[w_d^3]  Denominator=[1 w_d]
  Transfer Fcn1 : TransferFcn  Denominator=[1 0]
  Transfer Fcn2 : TransferFcn  Denominator=[1 0]
  y_filtered : Outport
  y_dot_d : Outport  Port=2
  y_ddot_d : Outport  Port=3
  wires:
  Transfer Fcn/1 -> Sum/1
  Transfer Fcn1/1 -> Saturation/1
  Sum1/1 -> y_ddot_d/1, Transfer Fcn1/1
  Saturation/1 -> y_dot_d/1, Gain/1, Transfer Fcn2/1
  Gain1/1 -> Sum/2
  Sum/1 -> Sum1/1
  Transfer Fcn2/1 -> y_filtered/1, Gain1/1
  Gain/1 -> Sum1/2
  y_ref (m)/1 -> Transfer Fcn/1

== system ASMC_sim_CSEI_FTESO/Enabled ESO Subsystem/ESO/Rotation_from Body2NED ==
  psi_rad : Inport
  MATLAB Function : MATLAB Function  TreatAsAtomicUnit=on
  R : Outport
  wires:
  psi_rad/1 -> MATLAB Function/1(psi)
  MATLAB Function/1(R) -> R/1

== system ASMC_sim_CSEI_FTESO/Enabled FTESO Subsystem/FTESO/Rotation_from Body2NED ==
  psi_rad : Inport
  MATLAB Function : MATLAB Function  TreatAsAtomicUnit=on
  R : Outport
  wires:
  psi_rad/1 -> MATLAB Function/1(psi)
  MATLAB Function/1(R) -> R/1

== matlab function ASMC_sim_CSEI_FTESO/CSEI ==
  data: xdot output; x input; tau input; current input; ME output; CE output; DE output; GE output; disturbance input
function [xdot, ME, CE, DE, GE]  = CSEI(x, tau, current, disturbance)
%% nu = [u, v, r], eta = [x, y, psi]
%  u:     surge velocity          (m/s)
%  v:     sway velocity           (m/s)
%  r:     yaw velocity            (rad/s)
%  x:     position in x direction (m)
%  y:     position in y direction (m)
%  psi:   yaw angle               (rad)

% This block calculates the change in position and heading given the
% current position and heading and velocities.


% State and current variables
nu = x(1:3); eta = x(4:6);
%% Initializing parameters
R = [cos(eta(3)) -sin(eta(3)) 0;
     sin(eta(3)) cos(eta(3)) 0;
     0 0 1];                        % Rotation matrix with heading
nu_c = R'*[current;0];              % Current velocity vector in body frame
nu_r = nu-nu_c;                     % Relative velocity
u   = nu_r(1);                      % Speed in x
v   = nu_r(2);                      % Speed in y
r   = nu_r(3);                      % Yaw rate

tau = [tau(1);tau(2);tau(3)] + [disturbance(1); disturbance(2); disturbance(3)];

%% MATRICES 
m    = 14.11;   I_z  =  1.7600;   x_g = 0.0375;

%% Added mass
X_ud  =     -2.0;											
					Y_vd =      -10.0;	N_vd =    -0.0;		
					Y_rd =      -0.0;	N_rd =    -1.0;	

%% Total mass matrix
m_11 = m-X_ud;
m_22 = m-Y_vd;
m_23 = m*x_g-Y_rd;
m_32 = m*x_g-N_vd;
m_33 = I_z-N_rd;

M    = [m_11 0    0
        0    m_22 m_23
        0    m_32 m_33];
	
%% Damping coefficients
% Comments at the end of the lines indicate the old values used.
X_u		= -0.6555;		X_v		= 0;
X_uu 	= 0.3545;		X_vv	= -2.443;
X_uuu 	= -3.787;		X_vvv	= 0;

						Y_v		= -1.33; 			Y_r		= -7.250; 
						Y_vv	= -2.776;			Y_rr	= -3.450; 
						Y_vvv	= -64.91;			Y_rrr	= 0;
						
						Y_rv	= -0.805;			Y_vr	= -0.845;

						N_v		= 0;				N_r		= -1.900;
						N_vv	= -0.2088;			N_rr	= -0.750;
						N_vvv	= 0;				N_rrr	= 0;
						
						N_rv	= 0.130;			N_vr	= 0.080;

%% Correolis matrix
c_13 = -(m-Y_vd)*v-(m*x_g-Y_rd)*r;
c_23 = (m-X_ud)*u;
C    = [0     0     c_13
        0     0     c_23
        -c_13 -c_23 0   ];

%% Assembly of the damping matrix
d_11 = -X_u - X_uu*u - X_uuu*u^2;
d_22 = -Y_v - Y_vv*v - Y_vvv*v^2 - Y_rv*abs(r);
d_33 = -N_r - N_rr*abs(r) - N_rrr*r^2 - N_vr*abs(v);

d_12 = -X_v - X_vv*v - X_vvv*v^2;
d_23 = -Y_r - Y_rr*abs(r) - Y_rrr*r^2 - Y_vr*abs(v);
d_32 = -N_v - N_vv*v - N_vvv*v^2 - N_rv*abs(r);

D    = [d_11 0 0
        0    d_22 d_23
        0    d_32 d_33];

%% Initializing
psi = eta(3);                       % Heading
R = [cos(psi) -sin(psi) 0
     sin(psi) cos(psi)  0
     0        0         1];         % Rotation matrix with heading
 
%% Calculating
eta_dot = R*(nu);
%% CALCULATION
nu_dot = M\(tau-(C+D)*nu_r);
tau_curr = (C+D)*nu_c;
xdot = [nu_dot;  % u, v, r
        eta_dot]; % x, y, psi

R_diff = [-sin(psi)*r -cos(psi)*r  0;
           cos(psi)*r  -sin(psi)*r  0;
           0         0         0];
inv_R = [ cos(psi), sin(psi), 0;
        -sin(psi), cos(psi), 0;
          0, 0, 1];                 
ME = R*M*inv_R;
CE = R*(C-M*inv_R*R_diff)*inv_R;
DE = R*D*inv_R;
GE = 0;
end

== matlab function ASMC_sim_CSEI_FTESO/ASMC/MATLAB Function1 ==
  data: tau_NED input; tau_Body output; psi input
function tau_Body = Coordinate_Conversion(tau_NED, psi)

R = [cos(psi), -sin(psi), 0;
     sin(psi), cos(psi), 0;
      0, 0, 1];

tau_Body = inv(R)*tau_NED;

== matlab function ASMC_sim_CSEI_FTESO/control allocation/Thruster modeling/MATLAB Function ==
  data: x1 output size=1; y1 output size=1; u_1 input size=1; a_1 input size=1; moment1 output size=1; f_VSP1_max input
function [x1,y1,moment1] = fcn(u_1, a_1, f_VSP1_max)
% This function takes in the input to VSP1 and calculates the resulting
% forces and moment.
    ly_VSP = 0.055;                         % Moment arm along y
    lx_VSP = 0.4574;                        % Moment arm along x
%     f_VSP1_max = 0.45;                      % Max thrust available
%     f_VSP1_max = 2.5;                      % Max thrust available

x1 = u_1*f_VSP1_max*cos(a_1);               % Resulting forces in x
y1 = u_1*f_VSP1_max*sin(a_1);               % Resulting forces in y
moment1 = x1*ly_VSP*(1) + y1*lx_VSP*(-1);   % Resulting moment

== matlab function ASMC_sim_CSEI_FTESO/Enabled FTESO Subsystem/FTESO/Matrix ==
  data: x1_hat input; x2_hat input; current input; ME output; CE output; DE output; GE output
function [ME, CE, DE, GE]  = CSEI(x1_hat, x2_hat, current)
%% nu = [u, v, r], eta = [x, y, psi]
%  u:     surge velocity          (m/s)
%  v:     sway velocity           (m/s)
%  r:     yaw velocity            (rad/s)
%  x:     position in x direction (m)
%  y:     position in y direction (m)
%  psi:   yaw angle               (rad)

% This block calculates the change in position and heading given the
% current position and heading and velocities.

% State and current variables
eta = x1_hat; % [x, y, psi]
eta_dot = x2_hat; % [x_dot, y_dot, psi_dot]

%% Initializing parameters
R = [cos(eta(3)) -sin(eta(3)) 0;
     sin(eta(3)) cos(eta(3)) 0;
     0 0 1];                        % Rotation matrix with heading

nu = R'*eta_dot;

nu_c = R'*[current;0];              % Current velocity vector in body frame
nu_r = nu-nu_c;                     % Relative velocity
u   = nu_r(1);                      % Speed in x
v   = nu_r(2);                      % Speed in y
r   = nu_r(3);                      % Yaw rate
%% MATRICES 
m    = 14.11;   I_z  =  1.7600;   x_g = 0.0375;

%% Added mass
X_ud  =     -2.0;											
					Y_vd =      -10.0;	N_vd =    -0.0;		
					Y_rd =      -0.0;	N_rd =    -1.0;	

%% Total mass matrix
m_11 = m-X_ud;
m_22 = m-Y_vd;
m_23 = m*x_g-Y_rd;
m_32 = m*x_g-N_vd;
m_33 = I_z-N_rd;

M    = [m_11 0    0
        0    m_22 m_23
        0    m_32 m_33];
	
%% Damping coefficients
% Comments at the end of the lines indicate the old values used.
X_u		= -0.6555;		X_v		= 0;
X_uu 	= 0.3545;		X_vv	= -2.443;
X_uuu 	= -3.787;		X_vvv	= 0;

						Y_v		= -1.33; 			Y_r		= -7.250; 
						Y_vv	= -2.776;			Y_rr	= -3.450; 
						Y_vvv	= -64.91;			Y_rrr	= 0;
						
						Y_rv	= -0.805;			Y_vr	= -0.845;

						N_v		= 0;				N_r		= -1.900;
						N_vv	= -0.2088;			N_rr	= -0.750;
						N_vvv	= 0;				N_rrr	= 0;
						
						N_rv	= 0.130;			N_vr	= 0.080;

%% Correolis matrix
c_13 = -(m-Y_vd)*v-(m*x_g-Y_rd)*r;
c_23 = (m-X_ud)*u;
C    = [0     0     c_13
        0     0     c_23
        -c_13 -c_23 0   ];

%% Assembly of the damping matrix
d_11 = -X_u - X_uu*u - X_uuu*u^2;
d_22 = -Y_v - Y_vv*v - Y_vvv*v^2 - Y_rv*abs(r);
d_33 = -N_r - N_rr*abs(r) - N_rrr*r^2 - N_vr*abs(v);

d_12 = -X_v - X_vv*v - X_vvv*v^2;
d_23 = -Y_r - Y_rr*abs(r) - Y_rrr*r^2 - Y_vr*abs(v);
d_32 = -N_v - N_vv*v - N_vvv*v^2 - N_rv*abs(r);

D    = [d_11 0 0
        0    d_22 d_23
        0    d_32 d_33];

%% Initializing
psi = eta(3);                       % Heading
R = [cos(psi) -sin(psi) 0
     sin(psi) cos(psi)  0
     0        0         1];         % Rotation matrix with heading
 
R_diff = [-sin(psi)*r -cos(psi)*r  0;
           cos(psi)*r  -sin(psi)*r  0;
           0         0         0];
inv_R = [ cos(psi), sin(psi), 0;
        -sin(psi), cos(psi), 0;
          0, 0, 1];                 
ME = R*M*inv_R;
CE = R*(C-M*inv_R*R_diff)*inv_R;
DE = R*D*inv_R;
GE = 0;
end

== matlab function ASMC_sim_CSEI_FTESO/Enabled FTESO Subsystem/FTESO/Rotation_from Body2NED/MATLAB Function ==
  data: psi input; R output
function R = Rotation_matrix(psi)

%% Initializing parameters
R = [cos(psi), -sin(psi), 0;
     sin(psi), cos(psi), 0;
     0, 0, 1];

== matlab function ASMC_sim_CSEI_FTESO/Enabled ESO Subsystem/ESO/ESO ==
  data: x_hat1 input; x_hat2 input; x_hat3 input; eta_dot input; x_hat1_dot output; x_hat2_dot output; tau_E input; x_hat3_dot output; x1 input; ME output; ME input; CE input; DE input; GE input; w0 input
function [x_hat1_dot, x_hat2_dot, x_hat3_dot, ME]  = ESO(x_hat1, x_hat2, x_hat3, eta_dot, tau_E, x1, ME,  CE, DE, GE, w0)
% xhat_1 = [x, y, psi]
% xhat_2 = [x_dot, y_dot, psi_dot]
% nu = [u, v, r];
% eta_dot = inv(ME)*z_hat1;


l0 = 3*w0*eye(3,3);
l1 = 3*w0^2*eye(3,3);
l2 = w0^3*eye(3,3);

input = -inv(ME)*(CE*eta_dot+DE*eta_dot+GE-tau_E);

x_hat1_dot = x_hat2 +l0*(x1-x_hat1);
x_hat2_dot = x_hat3 +l1*(x1-x_hat1) + input ;
x_hat3_dot = l2*(x1-x_hat1);

== matlab function ASMC_sim_CSEI_FTESO/control allocation/Thruster modeling/MATLAB Function1 ==
  data: x2 output size=1; u_2 input size=1; y2 output size=1; a_2 input size=1; moment2 output size=1; f_VSP2_max input
function [x2,y2,moment2] = fcn(u_2,a_2, f_VSP2_max)
% This function takes in the input to VSP2 and calculates the resulting
% forces and moment.
    ly_VSP = 0.055;                         % Moment arm along y
    lx_VSP = 0.4574;                        % Moment arm along x
%     f_VSP2_max = 0.45;                      % Max thrust available
%     f_VSP2_max = 2.5;                      % Max thrust available

x2 = u_2*f_VSP2_max*cos(a_2);               % Resulting forces in x
y2 = u_2*f_VSP2_max*sin(a_2);               % Resulting forces in y
moment2 = x2*ly_VSP*(-1) + y2*lx_VSP*(-1);  % Resulting moment

== matlab function ASMC_sim_CSEI_FTESO/control allocation/Thruster modeling/MATLAB Function2 ==
  data: u_bt input size=1; y3 output size=1; moment3 output size=1; f_BT_max input
function [y3,moment3] = fcn(u_bt, f_BT_max)
% This function takes in the input to the BT and calculates the resulting
% forces and moment.
    lx_BT = 0.3875;         % Moment arm along x
%     f_BT_max = 0.3;         % Max thrust available
%     f_BT_max = 2;         % Max thrust available
    
    y3 = u_bt*f_BT_max;     % Resulting force in y
    moment3 = y3*lx_BT;     % Resulting moment

== matlab function ASMC_sim_CSEI_FTESO/Enabled ESO Subsystem/ESO/Matrix ==
  data: x1_hat input; x2_hat input; current input; ME output; CE output; DE output; GE output
function [ME, CE, DE, GE]  = CSEI(x1_hat, x2_hat, current)
%% nu = [u, v, r], eta = [x, y, psi]
%  u:     surge velocity          (m/s)
%  v:     sway velocity           (m/s)
%  r:     yaw velocity            (rad/s)
%  x:     position in x direction (m)
%  y:     position in y direction (m)
%  psi:   yaw angle               (rad)

% This block calculates the change in position and heading given the
% current position and heading and velocities.

% State and current variables
eta = x1_hat; % [x, y, psi]
eta_dot = x2_hat; % [x_dot, y_dot, psi_dot]

%% Initializing parameters
R = [cos(eta(3)) -sin(eta(3)) 0;
     sin(eta(3)) cos(eta(3)) 0;
     0 0 1];                        % Rotation matrix with heading

nu = R'*eta_dot;

nu_c = R'*[current;0];              % Current velocity vector in body frame
nu_r = nu-nu_c;                     % Relative velocity
u   = nu_r(1);                      % Speed in x
v   = nu_r(2);                      % Speed in y
r   = nu_r(3);                      % Yaw rate
%% MATRICES 
m    = 14.11;   I_z  =  1.7600;   x_g = 0.0375;

%% Added mass
X_ud  =     -2.0;											
					Y_vd =      -10.0;	N_vd =    -0.0;		
					Y_rd =      -0.0;	N_rd =    -1.0;	

%% Total mass matrix
m_11 = m-X_ud;
m_22 = m-Y_vd;
m_23 = m*x_g-Y_rd;
m_32 = m*x_g-N_vd;
m_33 = I_z-N_rd;

M    = [m_11 0    0
        0    m_22 m_23
        0    m_32 m_33];
	
%% Damping coefficients
% Comments at the end of the lines indicate the old values used.
X_u		= -0.6555;		X_v		= 0;
X_uu 	= 0.3545;		X_vv	= -2.443;
X_uuu 	= -3.787;		X_vvv	= 0;

						Y_v		= -1.33; 			Y_r		= -7.250; 
						Y_vv	= -2.776;			Y_rr	= -3.450; 
						Y_vvv	= -64.91;			Y_rrr	= 0;
						
						Y_rv	= -0.805;			Y_vr	= -0.845;

						N_v		= 0;				N_r		= -1.900;
						N_vv	= -0.2088;			N_rr	= -0.750;
						N_vvv	= 0;				N_rrr	= 0;
						
						N_rv	= 0.130;			N_vr	= 0.080;

%% Correolis matrix
c_13 = -(m-Y_vd)*v-(m*x_g-Y_rd)*r;
c_23 = (m-X_ud)*u;
C    = [0     0     c_13
        0     0     c_23
        -c_13 -c_23 0   ];

%% Assembly of the damping matrix
d_11 = -X_u - X_uu*u - X_uuu*u^2;
d_22 = -Y_v - Y_vv*v - Y_vvv*v^2 - Y_rv*abs(r);
d_33 = -N_r - N_rr*abs(r) - N_rrr*r^2 - N_vr*abs(v);

d_12 = -X_v - X_vv*v - X_vvv*v^2;
d_23 = -Y_r - Y_rr*abs(r) - Y_rrr*r^2 - Y_vr*abs(v);
d_32 = -N_v - N_vv*v - N_vvv*v^2 - N_rv*abs(r);

D    = [d_11 0 0
        0    d_22 d_23
        0    d_32 d_33];

%% Initializing
psi = eta(3);                       % Heading
R = [cos(psi) -sin(psi) 0
     sin(psi) cos(psi)  0
     0        0         1];         % Rotation matrix with heading
 
R_diff = [-sin(psi)*r -cos(psi)*r  0;
           cos(psi)*r  -sin(psi)*r  0;
           0         0         0];
inv_R = [ cos(psi), sin(psi), 0;
        -sin(psi), cos(psi), 0;
          0, 0, 1];                 
ME = R*M*inv_R;
CE = R*(C-M*inv_R*R_diff)*inv_R;
DE = R*D*inv_R;
GE = 0;
end

== matlab function ASMC_sim_CSEI_FTESO/Enabled ESO Subsystem/ESO/Rotation_from Body2NED/MATLAB Function ==
  data: psi input; R output
function R = Rotation_matrix(psi)

%% Initializing parameters
R = [cos(psi), -sin(psi), 0;
     sin(psi), cos(psi), 0;
     0, 0, 1];

== matlab function ASMC_sim_CSEI_FTESO/Subsystem/MATLAB Function1 ==
  data: psi input; psi_mod output
function psi_mod = wrapToPi(psi)

psi_mod = mod(psi + pi, 2*pi) - pi;

== matlab function ASMC_sim_CSEI_FTESO/Subsystem1/MATLAB Function1 ==
  data: psi input; psi_mod output
function psi_mod = wrapToPi(psi)

psi_mod = mod(psi + pi, 2*pi) - pi;

== matlab function ASMC_sim_CSEI_FTESO/ASMC/k1 adaptive gain ==
  data: k1_dot output; s input; mu input; k1 input; k3 input; k_min input
function k1_dot = ASMC_k1(s, mu, k1, k3, k_min)

k1_dot = [0;0;0];
persistent firstRun

if isempty(firstRun)
    firstRun = 1;
    k1 = [1;1;1];
end

if k1(1) > k_min
    k1_dot(1) = k3(1)*sign(abs(s(1))-mu(1));
elseif k1(1) <= k_min
    k1_dot(1) = k_min;
end

if k1(2) > k_min
    k1_dot(2) = k3(2)*sign(abs(s(2))-mu(2));
elseif k1(2) <= k_min
    k1_dot(2) = k_min;
end


if k1(3) > k_min
    k1_dot(3) = k3(3)*sign(abs(s(3))-mu(3));
elseif k1(3) <= k_min
    k1_dot(3) = k_min;
end

== matlab function ASMC_sim_CSEI_FTESO/ASMC/ASMC ==
  data: s input; k1 input; k2 input; tau_a output
function tau_a = ASMC(s, k1 , k2)

tau_a = k1.*sqrt(abs(s)).*sign(s)+k2.*s;

== matlab function ASMC_sim_CSEI_FTESO/Enabled FTESO Subsystem/FTESO/FTESO ==
  data: x_hat1 input; x_hat2 input; x_hat3 input; eta_dot input; x_hat1_dot output; x_hat2_dot output; tau_E input; x_hat3_dot output; x1 input; ME output; ME input; CE input; DE input; GE input; w0 input
function [x_hat1_dot, x_hat2_dot, x_hat3_dot, ME]  = FTESO(x_hat1, x_hat2, x_hat3, eta_dot, tau_E, x1, ME,  CE, DE, GE, w0)
% xhat_1 = [x, y, psi]
% xhat_2 = [x_dot, y_dot, psi_dot]
% nu = [u, v, r];
% eta_dot = inv(ME)*z_hat1;


l0 = 3*w0*eye(3,3);
l1 = 3*w0^2*eye(3,3);
l2 = w0^3*eye(3,3);
alpha = 0.8;

input = -inv(ME)*(CE*eta_dot+DE*eta_dot+GE-tau_E);

x_hat1_dot = x_hat2 +l0*abs(x1-x_hat1).^((alpha+1)/2).*sign(x1-x_hat1);
x_hat2_dot = x_hat3 +l1*abs(x1-x_hat1).^((alpha+1)/2).*sign(x1-x_hat1) + input ;
x_hat3_dot = l2*abs(x1-x_hat1).^alpha.*sign(x1-x_hat1);
